simulink subsystem "MotoresN20"  (R2025a)
settings: Solver=VariableStepAuto  StartTime=0.0  StopTime=10.0  RelTol=1e-3
libraries: arduinolib x8
settings Model: Creator=Antonio  LastModifiedBy=aj
settings RTWCC: GPUComputeCapability=3.5

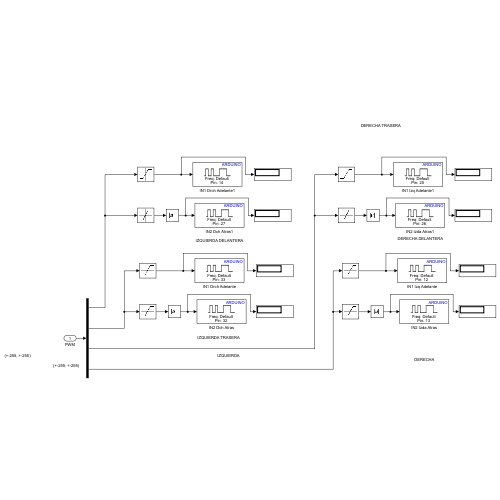
[thumbnail: Simulink's stored preview of the top-level diagram]
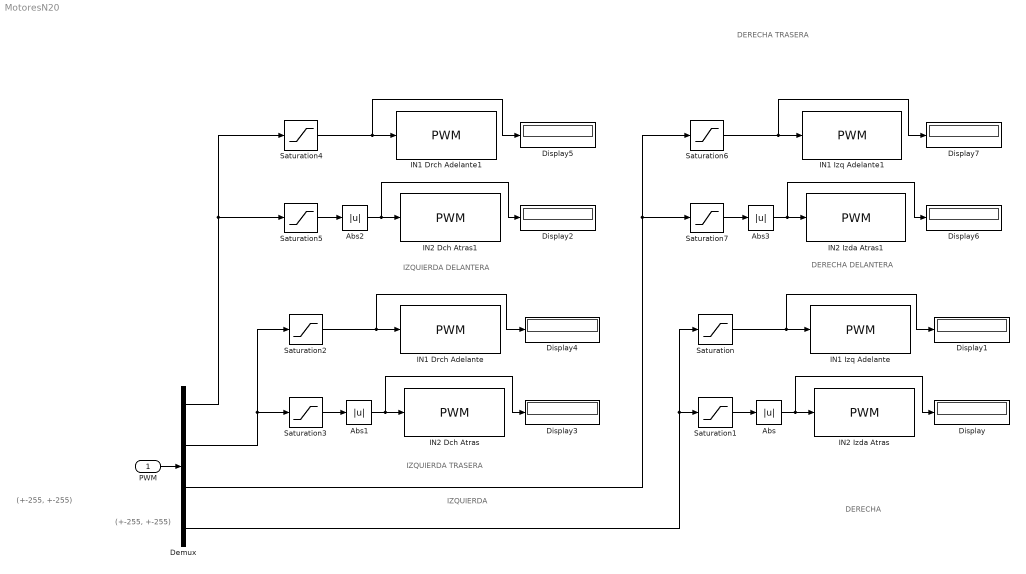
== system MotoresN20 ==
  note: DERECHA
  note: IZQUIERDA
  note: (+-255, +-255)
  note: (+-255, +-255)
  note: DERECHA DELANTERA
  note: IZQUIERDA DELANTERA
  note: DERECHA TRASERA
  note: IZQUIERDA TRASERA
  PWM : Inport
  Abs{,1..3} (4 alike) : Abs  SaturateOnIntegerOverflow=off
  Demux : Demux
  Display{,1..7} (8 alike) : Display
  IN1 Drch Adelante : arduinolib/PWM  pinNumber=33  frequencyType=Default  desiredFrequency=490.2  achievableFrequency=490.2
  IN1 Drch Adelante1 : arduinolib/PWM  pinNumber=14  frequencyType=Default  desiredFrequency=490.2  achievableFrequency=490.2
  IN1 Izq Adelante : arduinolib/PWM  pinNumber=12  frequencyType=Default  desiredFrequency=490.2  achievableFrequency=490.2
  IN1 Izq Adelante1 : arduinolib/PWM  pinNumber=25  frequencyType=Default  desiredFrequency=490.2  achievableFrequency=490.2
  IN2 Dch Atras : arduinolib/PWM  pinNumber=32  frequencyType=Default  desiredFrequency=490.2  achievableFrequency=490.2
  IN2 Dch Atras1 : arduinolib/PWM  pinNumber=27  frequencyType=Default  desiredFrequency=490.2  achievableFrequency=490.2
  IN2 Izda Atras : arduinolib/PWM  pinNumber=13  frequencyType=Default  desiredFrequency=490.2  achievableFrequency=490.2
  IN2 Izda Atras1 : arduinolib/PWM  pinNumber=26  frequencyType=Default  desiredFrequency=490.2  achievableFrequency=490.2
  Saturation{,2,4,6} (4 alike) : Saturate  UpperLimit=255  LowerLimit=1
  Saturation{1,3,5,7} (4 alike) : Saturate  UpperLimit=0  LowerLimit=-255
  wires:
  PWM/1 -> Demux/1
  Saturation6/1 -> IN1 Izq Adelante1/1, Display7/1
  Saturation/1 -> IN1 Izq Adelante/1, Display1/1
  Saturation1/1 -> Abs/1
  Saturation4/1 -> Display5/1, IN1 Drch Adelante1/1
  Abs1/1 -> IN2 Dch Atras/1, Display3/1
  Abs3/1 -> Display6/1, IN2 Izda Atras1/1
  Abs2/1 -> IN2 Dch Atras1/1, Display2/1
  Demux/4 -> Saturation1/1, Saturation/1
  Abs/1 -> Display/1, IN2 Izda Atras/1
  Saturation5/1 -> Abs2/1
  Saturation2/1 -> Display4/1, IN1 Drch Adelante/1
  Saturation3/1 -> Abs1/1
  Demux/1 -> Saturation5/1, Saturation4/1
  Demux/2 -> Saturation3/1, Saturation2/1
  Saturation7/1 -> Abs3/1
  Demux/3 -> Saturation6/1, Saturation7/1
